simulink model "PS3_out"  (R2016b)
settings: Solver=VariableStepAuto  StartTime=0.0  StopTime=20  RelTol=1e-3
libraries: vrlib x1
settings Model: Creator=Ørjan  LastModifiedBy=Ørjan

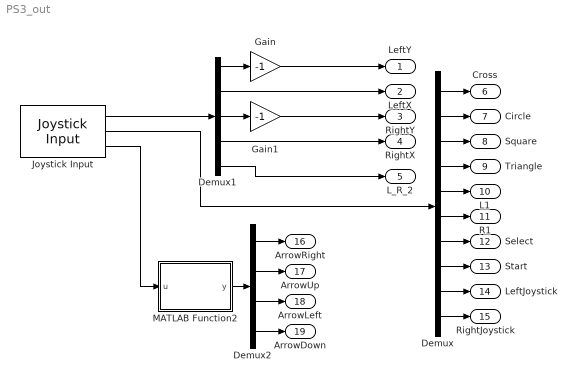
== system PS3_out ==
  Demux : Demux  Outputs=10
  Demux1 : Demux  Outputs=5
  Demux2 : Demux
  Gain : Gain  Gain=-1
  Gain1 : Gain  Gain=-1
  Joystick Input : vrlib/Joystick Input  joyid=1  adjustports=on  forcefeed=off
  MATLAB Function2 : MATLAB Function  TreatAsAtomicUnit=on
  LeftY : Outport
  LeftX : Outport  Port=2
  RightY : Outport  Port=3
  RightX : Outport  Port=4
  L_R_2 : Outport  Port=5
  Cross : Outport  Port=6
  Circle : Outport  Port=7
  Square : Outport  Port=8
  Triangle : Outport  Port=9
  L1 : Outport  Port=10
  R1 : Outport  Port=11
  Select : Outport  Port=12
  Start : Outport  Port=13
  LeftJoystick : Outport  Port=14
  RightJoystick : Outport  Port=15
  ArrowRight : Outport  Port=16
  ArrowUp : Outport  Port=17
  ArrowLeft : Outport  Port=18
  ArrowDown : Outport  Port=19
  wires:
  Joystick Input/1 -> Demux1/1
  Demux1/1 -> Gain/1
  Gain/1 -> LeftY/1
  Demux1/2 -> LeftX/1
  Demux1/3 -> Gain1/1
  Gain1/1 -> RightY/1
  Demux1/4 -> RightX/1
  Demux1/5 -> L_R_2/1
  Joystick Input/3 -> MATLAB Function2/1(u)
  Joystick Input/2 -> Demux/1
  Demux/1 -> Cross/1
  Demux/2 -> Circle/1
  Demux/3 -> Square/1
  Demux/4 -> Triangle/1
  Demux/5 -> L1/1
  Demux/6 -> R1/1
  Demux/7 -> Select/1
  Demux/8 -> Start/1
  Demux/9 -> LeftJoystick/1
  Demux/10 -> RightJoystick/1
  MATLAB Function2/1(y) -> Demux2/1
  Demux2/1 -> ArrowRight/1
  Demux2/2 -> ArrowUp/1
  Demux2/3 -> ArrowLeft/1
  Demux2/4 -> ArrowDown/1

== matlab function PS3_out/MATLAB Function2 ==
  data: u input; y output
function y = fcn(u)
    y = zeros(1, 4);
    switch u
        case 0
            y(1) = 1;
        case 90
            y(2) = 1;
        case 180
            y(3) = 1;
        case 270
            y(4) = 1;
    end
end
